simulink model "Troubleshooting_Engine_v4"  (R2013a)
settings: Solver=ode3  StartTime=0.0  StopTime=50  FixedStep=0.25  RelTol=1e-3
libraries: simulink x3
settings Model: Creator=Raymond  LastModifiedBy=Raymond

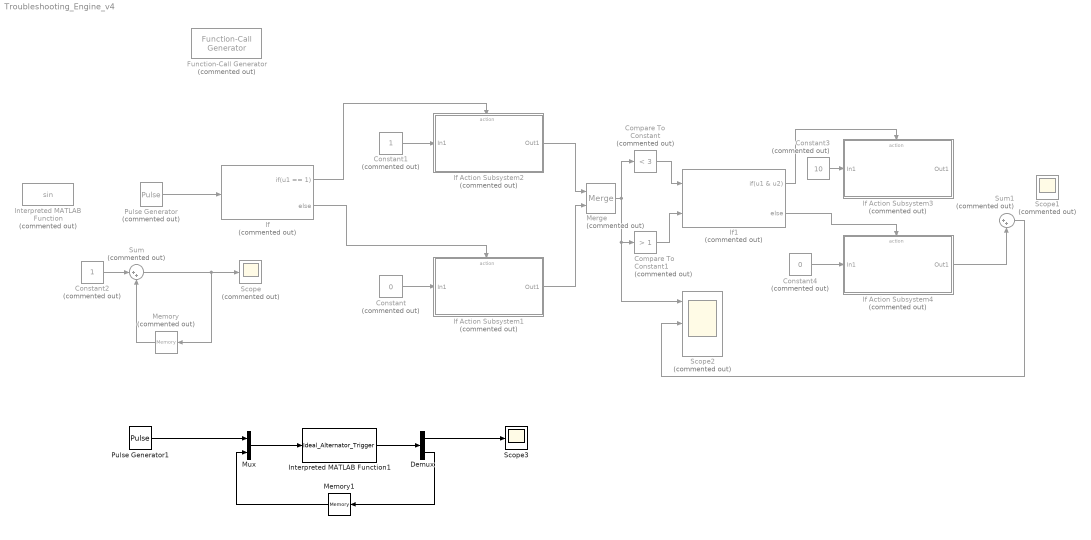
== system Troubleshooting_Engine_v4 ==
  Compare To Constant : simulink/Logic and Bit Operations/Compare To Constant  Commented=on  relop=<  const=3  OutDataTypeStr=boolean
  Compare To Constant1 : simulink/Logic and Bit Operations/Compare To Constant  Commented=on  relop=>  const=1  OutDataTypeStr=boolean
  Constant : Constant  Commented=on  Value=0
  Constant1 : Constant  Commented=on
  Constant2 : Constant  Commented=on
  Constant3 : Constant  Commented=on  Value=10
  Constant4 : Constant  Commented=on  Value=0
  Demux : Demux  Outputs=2
  Function-Call Generator : simulink/Ports & Subsystems/Function-Call Generator  Commented=on  sample_time=1  numberOfIterations=1
  If : If  Commented=on  IfExpression=u1 == 1
  If Action Subsystem1 : Subsystem  Commented=on  TreatAsAtomicUnit=on
  If Action Subsystem2 : Subsystem  Commented=on  TreatAsAtomicUnit=on
  If Action Subsystem3 : Subsystem  Commented=on  TreatAsAtomicUnit=on
  If Action Subsystem4 : Subsystem  Commented=on  TreatAsAtomicUnit=on
  If1 : If  Commented=on  NumInputs=2  IfExpression=u1 & u2
  Interpreted MATLAB Function : MATLABFcn  Commented=on
  Interpreted MATLAB Function1 : MATLABFcn  MATLABFcn=Ideal_Alternator_Trigger
  Memory : Memory  Commented=on
  Memory1 : Memory
  Merge : Merge  Commented=on
  Mux : Mux  Inputs=2
  Pulse Generator : DiscretePulseGenerator  Commented=on  PulseType=Time based  Period=5  PulseWidth=20
  Pulse Generator1 : DiscretePulseGenerator  PulseType=Time based  Period=5  PulseWidth=5
  Scope : Scope  Commented=on
  Scope1 : Scope  Commented=on
  Scope2 : Scope  Commented=on  NumInputPorts=3
      settings: YMin=-5~-5~-5  YMax=5~5~5  SaveName=ScopeData2
  Scope3 : Scope
      settings: SaveName=ScopeData3
  Sum : Sum  Commented=on  Inputs=|++
  Sum1 : Sum  Commented=on  Inputs=|++
  wires:
  If/1 -> If Action Subsystem2/Action
  If/2 -> If Action Subsystem1/Action
  If Action Subsystem2/1(Out1) -> Merge/1
  If Action Subsystem1/1(Out1) -> Merge/2
  Pulse Generator/1 -> If/1
  Constant/1 -> If Action Subsystem1/1(In1)
  Constant1/1 -> If Action Subsystem2/1(In1)
  Constant2/1 -> Sum/1
  Sum/1 -> Scope/1, Memory/1
  Memory/1 -> Sum/2
  Constant3/1 -> If Action Subsystem3/1(In1)
  Constant4/1 -> If Action Subsystem4/1(In1)
  If1/2 -> If Action Subsystem4/Action
  If Action Subsystem4/1(Out1) -> Sum1/2
  Sum1/1 -> Scope2/2
  Merge/1 -> Compare To Constant/1, Scope2/1, Compare To Constant1/1
  Compare To Constant/1 -> If1/1
  Compare To Constant1/1 -> If1/2
  If1/1 -> If Action Subsystem3/Action
  Pulse Generator1/1 -> Mux/1
  Interpreted MATLAB Function1/1 -> Demux/1
  Demux/1 -> Scope3/1
  Demux/2 -> Memory1/1
  Mux/1 -> Interpreted MATLAB Function1/1
  Memory1/1 -> Mux/2

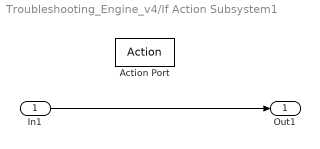
== system Troubleshooting_Engine_v4/If Action Subsystem1 ==
  In1 : Inport
  Action Port : ActionPort  ActionType=else
  Out1 : Outport
  wires:
  In1/1 -> Out1/1

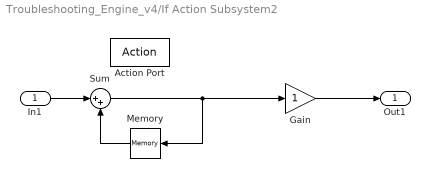
== system Troubleshooting_Engine_v4/If Action Subsystem2 ==
  In1 : Inport
  Action Port : ActionPort  ActionType=then
  Gain : Gain
  Memory : Memory
  Sum : Sum  Inputs=|++
  Out1 : Outport
  wires:
  In1/1 -> Sum/1
  Sum/1 -> Gain/1, Memory/1
  Memory/1 -> Sum/2
  Gain/1 -> Out1/1

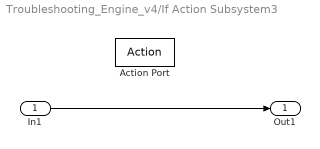
== system Troubleshooting_Engine_v4/If Action Subsystem3 ==
  In1 : Inport
  Action Port : ActionPort  ActionType=then
  Out1 : Outport
  wires:
  In1/1 -> Out1/1

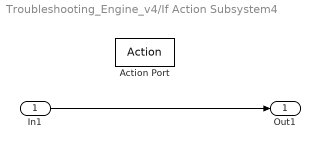
== system Troubleshooting_Engine_v4/If Action Subsystem4 ==
  In1 : Inport
  Action Port : ActionPort  ActionType=else
  Out1 : Outport
  wires:
  In1/1 -> Out1/1
